simulink model "Simple_source"  (R2018b)
settings: Solver=FixedStepDiscrete  StartTime=0.0  StopTime=10  FixedStep=Ts  RelTol=1e-3
PreLoadFcn:
  | setMatlabPaths
  | Ts = 1e-3
undefined symbols (not defined in the file or in its folder): sigbuilder_block
libraries: Simple_lib x9
settings Model: NumberOfSteps=100  Creator=billw  LastModifiedBy=billw

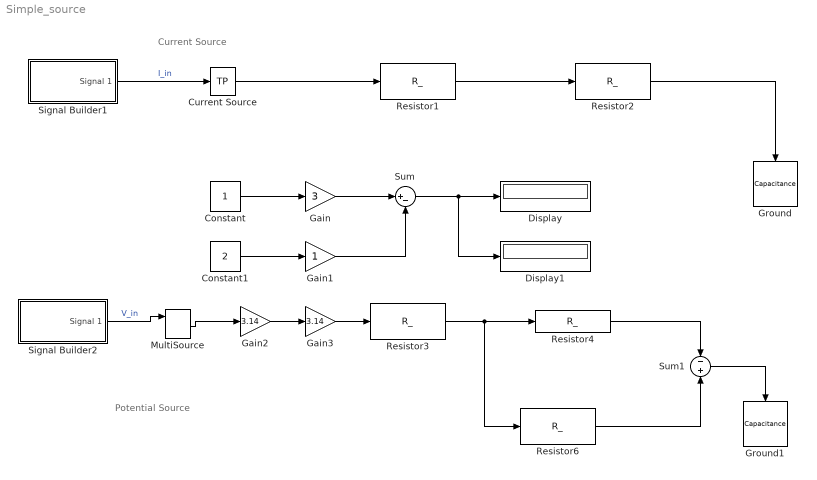
== system Simple_source ==
  note: Current Source
  note: Potential Source
  Constant : Constant
  Constant1 : Constant  Value=2
  Current Source : Simple_lib/Electronics/TP  V_0=0.0  slew_rate=inf  conserved_quantity_name=Q  energy_name=E
  Display : Display
  Display1 : Display
  Gain : Gain  Gain=3
  Gain1 : Gain
  Gain2 : Gain  Gain=3.14
  Gain3 : Gain  Gain=3.14
  Ground : Simple_lib/Electronics/Capacitance  C=inf
      settings: AttributesFormatString=%<C> F
  Ground1 : Simple_lib/Electronics/Capacitance  C=inf
      settings: AttributesFormatString=%<C> F
  MultiSource : Simple_lib/Electronics/MultiSource  V_0=inf  slew_rate=inf  conserved_quantity_name=Q  energy_name=E
  Resistor1 : Simple_lib/Electronics/R_  Exponent=3  R=1000
      link override at: slew_rate=inf
      settings: AttributesFormatString=%<R> Ohm
  Resistor2 : Simple_lib/Electronics/R_  Exponent=3  R=1000
      link override at: slew_rate=inf
      settings: AttributesFormatString=%<R> Ohm
  Resistor3 : Simple_lib/Electronics/R_  Exponent=0  R=1
      settings: AttributesFormatString=%<R> Ohm
  Resistor4 : Simple_lib/Electronics/R_  Exponent=2  R=100
      link override at: slew_rate=inf
      settings: AttributesFormatString=%<R> Ohm
  Resistor6 : Simple_lib/Electronics/R_  Exponent=4  R=10000
      settings: AttributesFormatString=%<R> Ohm
  Signal Builder1 : Subsystem  Tag=STV Subsys  LoadFcn=sigbuilder_block('load');  StartFcn=sigbuilder_block('start');  StopFcn=sigbuilder_block('stop');  ClipboardFcn=sigbuilder_block('clipboard');  mask(Sigbuilder block){tuvar=[0:10]}
      mask help: Simulink:masks:SigbuilderBlock_MD
      mask init:
      | if ~strcmp(get_param(bdroot(gcbh),'SimulationStatus'),'stopped') tuvar = sigbuilder_block('maskInit'); end
      settings: CopyFcn=sigbuilder_block('copy');  DeleteFcn=sigbuilder_block('delete');  ModelCloseFcn=sigbuilder_block('modelClose');  PreSaveFcn=sigbuilder_block('preSave');  PauseFcn=sigbuilder_block('pause');  ContinueFcn=sigbuilder_block('continue');  NameChangeFcn=sigbuilder_block('namechange');  OpenFcn=sigbuilder_block('open',[437.6 199.2 550.4 400 ]);  CloseFcn=sigbuilder_block('close');
      mask Display: plot(0, 0, 100, 100,[2, 2, 32, 32, 2], [68, 8, 8, 68, 68],[32, 2], [38, 38], [32, 19, 2],[53, 60, 44], [32, 17, 17, 2],[16, 16, 31, 31]);txt = getActiveGroup(gcbh);text(2, 100, txt,'verticalAlignment', 'top');
  Signal Builder2 : Subsystem  Tag=STV Subsys  LoadFcn=sigbuilder_block('load');  StartFcn=sigbuilder_block('start');  StopFcn=sigbuilder_block('stop');  ClipboardFcn=sigbuilder_block('clipboard');  mask(Sigbuilder block){tuvar=[0:10]}
      mask help: Simulink:masks:SigbuilderBlock_MD
      mask init:
      | if ~strcmp(get_param(bdroot(gcbh),'SimulationStatus'),'stopped') tuvar = sigbuilder_block('maskInit'); end
      settings: CopyFcn=sigbuilder_block('copy');  DeleteFcn=sigbuilder_block('delete');  ModelCloseFcn=sigbuilder_block('modelClose');  PreSaveFcn=sigbuilder_block('preSave');  PauseFcn=sigbuilder_block('pause');  ContinueFcn=sigbuilder_block('continue');  NameChangeFcn=sigbuilder_block('namechange');  OpenFcn=sigbuilder_block('open',[437.6 199.2 550.4 400 ]);  CloseFcn=sigbuilder_block('close');
      mask Display: plot(0, 0, 100, 100,[2, 2, 32, 32, 2], [68, 8, 8, 68, 68],[32, 2], [38, 38], [32, 19, 2],[53, 60, 44], [32, 17, 17, 2],[16, 16, 31, 31]);txt = getActiveGroup(gcbh);text(2, 100, txt,'verticalAlignment', 'top');
  Sum : Sum  Inputs=|+-
  Sum1 : Sum  Inputs=-|+
  wires:
  Resistor1/1 -> Resistor2/1
  Current Source/1 -> Resistor1/1
  Signal Builder1/1(Signal 1) -> Current Source/1  "I_in"
  Resistor2/1 -> Ground/1
  Signal Builder2/1(Signal 1) -> MultiSource/1  "V_in"
  MultiSource/1 -> Gain2/1
  Resistor3/1 -> Resistor6/1, Resistor4/1
  Resistor4/1 -> Sum1/1
  Sum/1 -> Display1/1, Display/1
  Constant/1 -> Gain/1
  Constant1/1 -> Gain1/1
  Gain/1 -> Sum/1
  Gain1/1 -> Sum/2
  Resistor6/1 -> Sum1/2
  Gain2/1 -> Gain3/1
  Gain3/1 -> Resistor3/1
  Sum1/1 -> Ground1/1

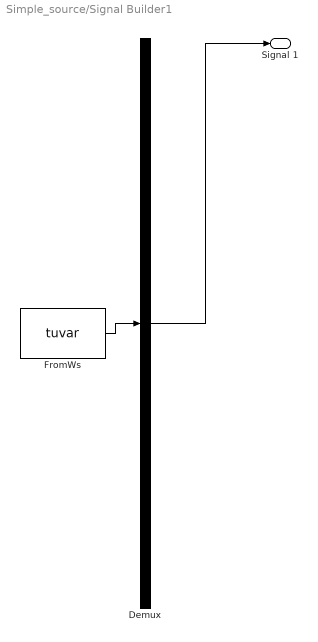
== system Simple_source/Signal Builder1 ==
  Demux : Demux  Tag=STV Demux  Outputs=1
  FromWs : FromWorkspace  Tag=STV FromWs  VariableName=tuvar  SampleTime=0
      SigBuilderData=|
      | common.afterFinalStr = 'Extrapolate'
      | common.sampleTime = 0
      | dataSet.timeRange = [0 10]
      | dataSet.name = 'Group 1'
      | sbobj.Groups.Name = 'Group 1'
      | sbobj.Groups.Signals.Name = 'Signal 1'
      | sbobj.Groups.Signals.XData = [0 4 4 6 6 10]
      | sbobj.Groups.Signals.YData = [0.39 0.39 1 1 0.225 0.225]
  Signal 1 : Outport  Tag=STV Outport
  wires:
  FromWs/1 -> Demux/1
  Demux/1 -> Signal 1/1

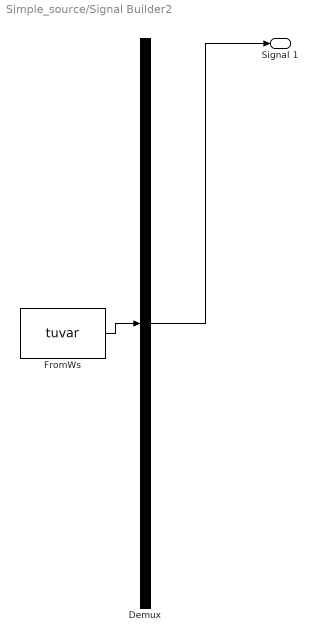
== system Simple_source/Signal Builder2 ==
  Demux : Demux  Tag=STV Demux  Outputs=1
  FromWs : FromWorkspace  Tag=STV FromWs  VariableName=tuvar  SampleTime=0
      SigBuilderData=|
      | common.afterFinalStr = 'Extrapolate'
      | common.sampleTime = 0
      | dataSet(1).timeRange = [0 10]
      | dataSet(1).name = 'Group 1'
      | dataSet(2).timeRange = [0 10]
      | dataSet(2).name = 'Group 2'
      | sbobj.Groups(1).Name = 'Group 1'
      | sbobj.Groups(1).Signals.Name = 'Signal 1'
      | sbobj.Groups(1).Signals.XData = [0 4 4 6 6 10]
      | sbobj.Groups(1).Signals.YData = [0.39 0.39 1 1 0.225 0.225]
      | sbobj.Groups(2).Name = 'Group 2'
      | sbobj.Groups(2).Signals.Name = 'Signal 1'
      | sbobj.Groups(2).Signals.XData = [0 0.125 0.25 0.375 0.5 0.625 0.75 0.875 1 1.125 1.25 1.375 1.5 1.625 1.75 1.875 2 2.125 2.25 2.375 2.5 2.625 2.75 2.875 3 3.125 3.25 3.375 3.5 3.625 3.75 3.875 4 4.125 4.25 4.375 4.5 4.625 4.75 4.875 5 5.125 5.25 5.375 5.5 5.625 5.75 5.875 6 6.125 6.25 6.375 6.5 6.625 6.75 6.875 7 7.125 7.25 7.375 7.5 7.625 7.75 7.875 8 8.125 8.25 8.375 8.5 8.625 8.75 8.875 9 9.125 9.25 9.375 9.5 9.625 9.75 9.875 10]
      | sbobj.Groups(2).Signals.YData = [1 1.70710678119 2 1.70710678119 1 0.292893218813 0 0.292893218813 1 1.70710678119 2 1.70710678119 1 0.292893218813 0 0.292893218813 1 1.70710678119 2 1.70710678119 1 0.292893218813 0 0.292893218813 1 1.70710678119 2 1.70710678119 1 0.292893218813 0 0.292893218813 1 1.70710678119 2 1.70710678119 1 0.292893218813 0 0.292893218813 1 1.70710678119 2 1.70710678119 1 0.292893218813 0 0.292893218813 1 1.70710678119 2 1.70710678119 1 0.292893218813 0 0.292893218813 1 1.70710678119 2 1.70710678119 1 0.292893218813 0 0.292893218813 1 1.70710678119 2 1.70710678119 1 0.292893218813 0 0.292893218813 1 1.70710678119 2 1.70710678119 1 0.292893218813 0 0.292893218813 1]
  Signal 1 : Outport  Tag=STV Outport
  wires:
  FromWs/1 -> Demux/1
  Demux/1 -> Signal 1/1
